simulink model "modFSKconst"  (Simulink 10.1)
settings: Solver=VariableStepAuto  StartTime=0.0  StopTime=10.0  RelTol=1e-3
undefined symbols (not defined in the file or in its folder): DiscIntNeverNeededParam
libraries: dspsrcs4 x2, commrandsrc3 x1, dspstat3 x1
settings Model: Creator=iba  LastModifiedBy=iba
settings DataIOCC: SaveFormat=Dataset  ReturnWorkspaceOutputs=on
settings OptimizationCC: LifeSpan=auto
settings DebuggingCC: UnderspecifiedInitializationDetection=Simplified  MergeDetectMultiDrivingBlocksExec=error  SFUnexpectedBacktrackingDiag=error  SFNoUnconditionalDefaultTransitionDiag=error  SFExecutionAtInitializationDiag=warning  ArithmeticOperatorsInVariantConditions=error
settings HardwareCC: ProdBitPerPointer=64  ProdBitPerSizeT=64  ProdBitPerPtrDiffT=64  ProdLargestAtomicFloat=Float  ProdIntDivRoundTo=Zero  ProdEndianess=LittleEndian  ProdWordSize=64  ProdHWDeviceType=Intel->x86-64 (Windows64)
settings ModelReferenceCC: PropagateSignalLabelsOutOfModel=on
settings SFSimCC: SimUseLocalCustomCode=on  CustomCodeUndefinedFunction=FilterOut
settings RTWCC: RTWUseLocalCustomCode=on
settings CodeAppCC: StateflowObjectComments=off
settings GRTTargetCC: TargetLangStandard=C99 (ISO)  CombineOutputUpdateFcns=on  GRTInterface=off
settings ConfigComp: CovMetricSettings=dwe  CovHtmlReporting=off  CovSaveCumulativeToWorkspaceVar=off  CovSaveSingleToWorkspaceVar=off  CovExternalEMLEnable=on

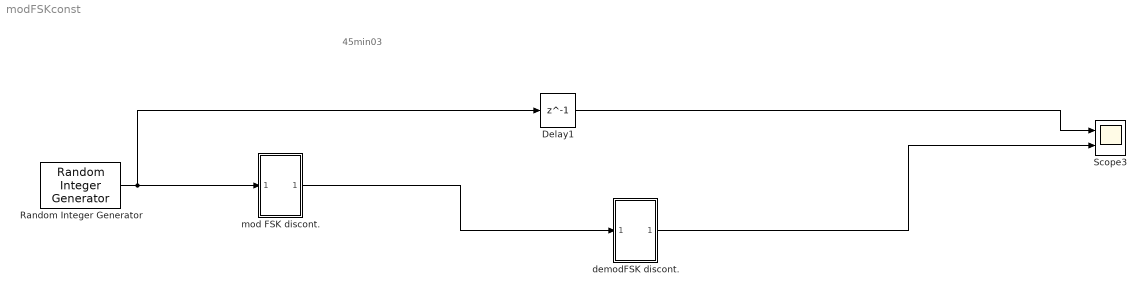
== system modFSKconst ==
  note: 45min03
  Delay1 : Delay  DelayLength=1  SampleTime=1
  Random Integer Generator : commrandsrc3/Random Integer Generator  SetSize=4  SeedSource=Parameter  Seed=37  SampleTime=1  SamplesPerFrame=1  OutputDataType=double  SimulateUsing=Interpreted execution
  Scope3 : Scope  NumInputPorts=2
  demodFSK discont. : Subsystem
  mod FSK discont. : Subsystem
  wires:
  Random Integer Generator/1 -> mod FSK discont./1(In1), Delay1/1
  Delay1/1 -> Scope3/1
  demodFSK discont./1(Out1) -> Scope3/2
  mod FSK discont./1(Out1) -> demodFSK discont./1(In1)

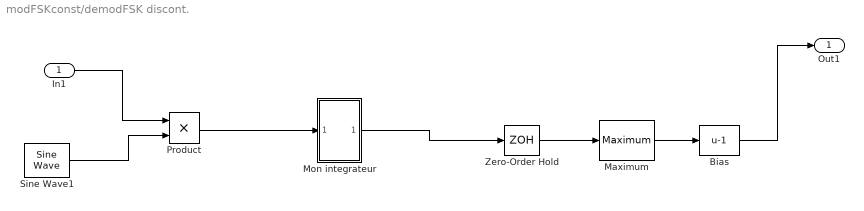
== system modFSKconst/demodFSK discont. ==
  In1 : Inport
  Bias : Bias  Bias=-1
  Maximum : dspstat3/Maximum  operation=maximum  fcn=Index  indexBase=Zero  operateOver=Entire input  Dimension=1  InputProcessing=Columns as channels (frame based)  reset=None  roiEnable=off  roiType=Rectangles  roiPortion=Entire ROI  roiOutput=Individual statistics for each ROI  roiFlag=off  roundingMode=Floor  overflowMode=off  accumDataTypeStr=Inherit: Same as product output  accumLastDataTypeStr=Inherit: Same as product output
  Mon integrateur : Subsystem
  Product : Product
  Sine Wave1 : dspsrcs4/Sine Wave  Amplitude=1  Frequency=(3:1.2:6.6)  Phase=0  SampleMode=Discrete  OutComplex=Real  CompMethod=Trigonometric fcn  TableSize=Speed  SampleTime=1/100  SamplesPerFrame=1  ResetState=Restart at time zero  OutputFrames=off  dataType=double  wordLen=16  udDataType=sfix(16)  fracBitsMode=Best precision  numFracBits=15  OutDataTypeStr=double  LastOutDataTypeStr=double
  Zero-Order Hold : ZeroOrderHold
  Out1 : Outport
  wires:
  Zero-Order Hold/1 -> Maximum/1
  Product/1 -> Mon integrateur/1(In1)
  Sine Wave1/1 -> Product/2
  Mon integrateur/1(Out1) -> Zero-Order Hold/1
  In1/1 -> Product/1
  Maximum/1 -> Bias/1
  Bias/1 -> Out1/1

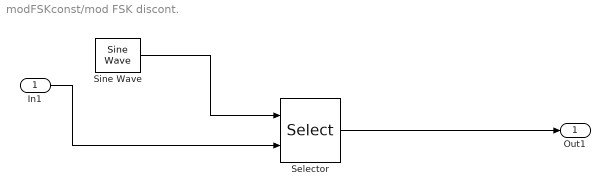
== system modFSKconst/mod FSK discont. ==
  In1 : Inport
  Selector : Selector  IndexMode=Zero-based  InputPortWidth=4  IndexOptions=Starting index (port)  Indices=[1 3]  OutputSizes=1
  Sine Wave : dspsrcs4/Sine Wave  Amplitude=1  Frequency=(3:1.2:6.6)  Phase=0  SampleMode=Discrete  OutComplex=Real  CompMethod=Trigonometric fcn  TableSize=Speed  SampleTime=1/100  SamplesPerFrame=1  ResetState=Restart at time zero  OutputFrames=off  dataType=double  wordLen=16  udDataType=sfix(16)  fracBitsMode=Best precision  numFracBits=15  OutDataTypeStr=double  LastOutDataTypeStr=double
  Out1 : Outport
  wires:
  In1/1 -> Selector/2
  Sine Wave/1 -> Selector/1
  Selector/1 -> Out1/1

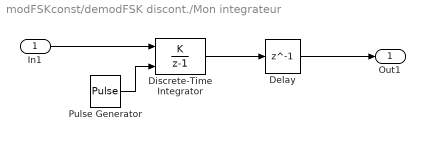
== system modFSKconst/demodFSK discont./Mon integrateur ==
  In1 : Inport
  Delay : Delay  DelayLength=1
  Discrete-Time Integrator : DiscreteIntegrator  IntegratorMethod=Accumulation: Forward Euler  ExternalReset=either  SampleTime=-1  ICPrevOutput=DiscIntNeverNeededParam  ICPrevScaledInput=DiscIntNeverNeededParam
  Pulse Generator : DiscretePulseGenerator
  Out1 : Outport
  wires:
  In1/1 -> Discrete-Time Integrator/1
  Pulse Generator/1 -> Discrete-Time Integrator/2
  Discrete-Time Integrator/1 -> Delay/1
  Delay/1 -> Out1/1
